simulink library "BLDC_controller_Lib_CounterBased"  (R2025a)
settings: Solver=VariableStepAuto  StartTime=0.0  StopTime=10.0  RelTol=1e-3
undefined symbols (not defined in the file): a_elecAngle, a_elecPeriod, a_phaAdv_M1, b_phaAdvEna, cf_speedCoef, cf_speedFilt, CTRL_COMM, n_commAcvLo, n_commDeacvHi, r_commDCDeacv, r_sin3PhaA_M1, r_sin3PhaB_M1, r_sin3PhaC_M1, r_sinPhaA_M1, r_sinPhaB_M1, r_sinPhaC_M1, r_trapPhaA_M1, r_trapPhaB_M1, r_trapPhaC_M1, vec_hallToPos, z_commutMap_M1, z_ctrlTypSel, z_hallDebSteps, z_maxCntRst, z_nrEdgeSpdAcv
libraries: BLDC_controller_Lib x4, simulink_extras x1, $bdroot x1, simulink x1, BLDC_controller_Lib_new x1
(part 1 of 2)
settings Model: Creator=37ef  LastModifiedBy=ernes
settings SolverCC: AlgebraicLoopSolver=TrustRegion
settings DataIOCC: ReturnWorkspaceOutputs=off
settings DebuggingCC: UnconnectedInputMsg=warning  UnconnectedOutputMsg=warning  UnconnectedLineMsg=warning  ArithmeticOperatorsInVariantConditions=warning
settings ModelReferenceCC: EnableRefExpFcnMdlSchedulingChecks=on
settings SFSimCC: SimUseLocalCustomCode=off  CustomCodeUndefinedFunction=UseInterfaceOnly
settings RTWCC: RTWUseLocalCustomCode=off  GPUComputeCapability=3.5

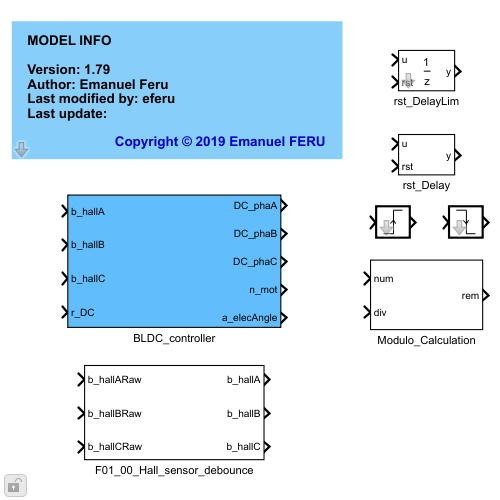
[thumbnail: Simulink's stored preview of the top-level diagram]
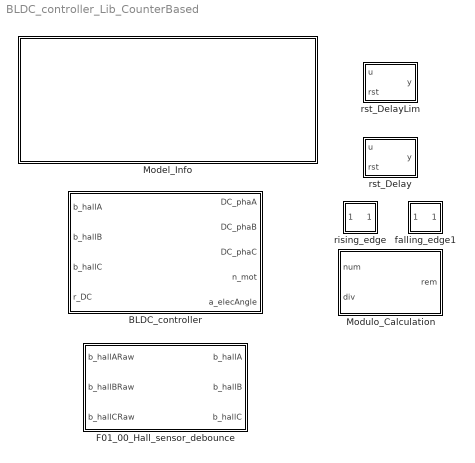
== system BLDC_controller_Lib_CounterBased ==
  BLDC_controller : Subsystem  SystemSampleTime=1e-5
  F01_00_Hall_sensor_debounce : Subsystem
  Model_Info : Subsystem
      mask DialogControl DescGroupVar Prompt: Model info
      mask DialogControl DescTextVar Prompt: This mask gives quick information about the model.
      mask Display:
      | info = Simulink.MDLInfo(bdroot);
      | file = dir([bdroot '.slx']);
      | % image('logo.png', [0.48, 0.55, 0.5, 0.4]);
      | text(0.05, 0.5, [...
      |         'MODEL INFO \n\n' ...
      |         'Version: ' info.ModelVersion '\n' ...
      |         'Author: ' 'Emanuel Feru' '\n' ...
      |         'Last modified by: ' info.LastModifiedBy '\n' ...
      |         'Last update: ' file.date '\n\n'], ...
      |         'horizontalAlignment', 'left', ...
      |         'verticalAlignment', 'middle');
      | 
      | color('blue');
      | text(0.95, 0.08, [...
      |         'Copyright © 2019 Emanuel FERU'], ...
      |         'horizontalAlignment', 'right', ...
      |         'verticalAlignment', 'bottom');
  Modulo_Calculation : Subsystem
  falling_edge1 : Subsystem  StopFcn=%tagged  TreatAsAtomicUnit=on  mask(Falling edge detection){}
      mask help:
      | Falling edge detection for a logic signal.
      | When a falling edge on the input signal is detected, the output switches to 1 during one time step.
      settings: RTWSystemCode=Nonreusable function
      mask Display: plot(0,0,100,100, [20 50 50 80], [90 90 10 10], [40 50 60], [55 45 55] )
  rising_edge : Subsystem  StopFcn=%tagged  TreatAsAtomicUnit=on  mask(Rising edge detection){}
      mask help:
      | Rising edge detection for a logic signal.
      | When a rising edge on the input signal is detected, the output switches to 1 during one time step.
      settings: RTWSystemCode=Nonreusable function
      mask Display: plot(0,0,100,100, [20 50 50 80], [10 10 90 90], [40 50 60], [45 55 45] )
  rst_Delay : Subsystem
  rst_DelayLim : Subsystem  mask{z_cntMaxLim=200}
      mask prompts: z_cntMaxLim "Maximum counter limit"
      mask Display: dpoly(1,[1 0],'z')

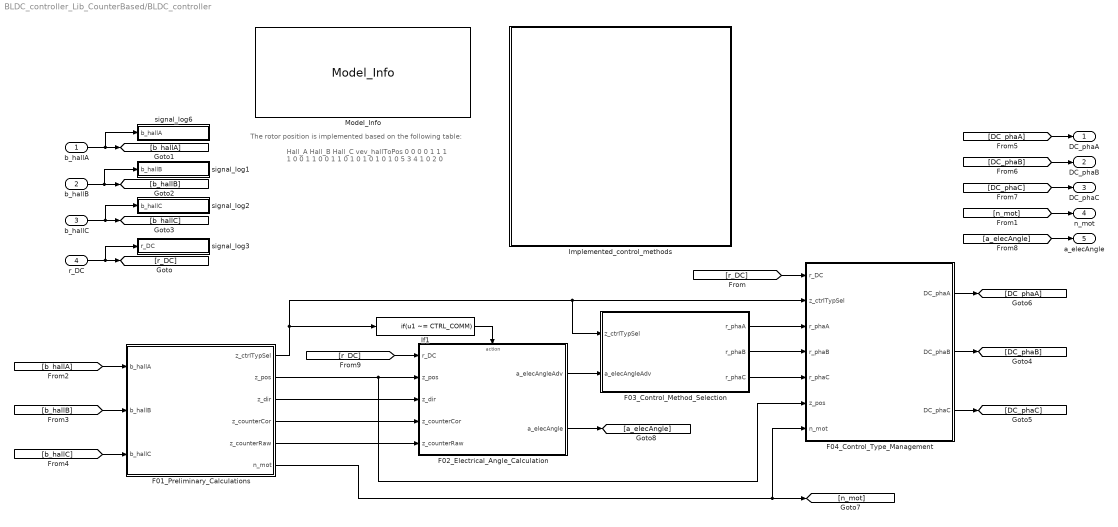
== system BLDC_controller_Lib_CounterBased/BLDC_controller ==
  note: Hall_A
      | Hall_B
      | Hall_C
      | vev_hallToPos
      |
      | 0
      | 0
      | 0
      | 0
      | 1
      | 1
      | 1
      | 1
      | 0
      | 0
      | 1
      | 1
      | 0
      | 0
      | 1
      | 1
      | 0
      | 1
      | 0
      | 1
      | 0
      | 1
      | 0
      | 1
      | 0
      | 5
      | 3
      | 4
      | 1
      | 0
      | 2
      | 0
  note: The rotor position is implemented based on the following table:
  "b_hallA " : Inport
  b_hallB : Inport  Port=2
  b_hallC : Inport  Port=3
  r_DC : Inport  Port=4
  F01_Preliminary_Calculations : Subsystem
  F02_Electrical_Angle_Calculation : Subsystem
  F03_Control_Method_Selection : Subsystem
  F04_Control_Type_Management : Subsystem
  If1 : If  IfExpression=u1 ~= CTRL_COMM  ShowElse=off
  Implemented_control_methods : Subsystem
      mask Display: image('control_methods.png')
  Model_Info : $bdroot/Model_Info
  signal_log1 : Subsystem
  signal_log2 : Subsystem
  signal_log3 : Subsystem
  signal_log6 : Subsystem
  DC_phaA : Outport  VectorParamsAs1DForOutWhenUnconnected=off
  DC_phaB : Outport  Port=2  VectorParamsAs1DForOutWhenUnconnected=off
  DC_phaC : Outport  Port=3  VectorParamsAs1DForOutWhenUnconnected=off
  n_mot : Outport  Port=4  VectorParamsAs1DForOutWhenUnconnected=off
  a_elecAngle : Outport  Port=5  VectorParamsAs1DForOutWhenUnconnected=off
  wires:
  [r_DC] -> F02_Electrical_Angle_Calculation/1(r_DC)
  F02_Electrical_Angle_Calculation/2(a_elecAngle) -> [a_elecAngle]
  [a_elecAngle] -> a_elecAngle/1
  r_DC/1 -> [r_DC], signal_log3/1(r_DC)
  [DC_phaC] -> DC_phaC/1
  [DC_phaB] -> DC_phaB/1
  F04_Control_Type_Management/3("DC_phaC ") -> [DC_phaC]
  F04_Control_Type_Management/2(DC_phaB) -> [DC_phaB]
  F04_Control_Type_Management/1(DC_phaA) -> [DC_phaA]
  [r_DC] -> F04_Control_Type_Management/1(r_DC)
  F03_Control_Method_Selection/3("r_phaC ") -> F04_Control_Type_Management/5(r_phaC)
  F03_Control_Method_Selection/2(r_phaB) -> F04_Control_Type_Management/4(r_phaB)
  F03_Control_Method_Selection/1(r_phaA) -> F04_Control_Type_Management/3(r_phaA)
  F02_Electrical_Angle_Calculation/1(a_elecAngleAdv) -> F03_Control_Method_Selection/2(a_elecAngleAdv)
  If1/1 -> F02_Electrical_Angle_Calculation/Action
  F01_Preliminary_Calculations/1(z_ctrlTypSel) -> If1/1, F03_Control_Method_Selection/1(z_ctrlTypSel), F04_Control_Type_Management/2(z_ctrlTypSel)
  F01_Preliminary_Calculations/5(z_counterRaw) -> F02_Electrical_Angle_Calculation/5(z_counterRaw)
  F01_Preliminary_Calculations/4(z_counterCor) -> F02_Electrical_Angle_Calculation/4(z_counterCor)
  F01_Preliminary_Calculations/6("n_mot ") -> [n_mot], F04_Control_Type_Management/7(n_mot)
  F01_Preliminary_Calculations/3(z_dir) -> F02_Electrical_Angle_Calculation/3(z_dir)
  F01_Preliminary_Calculations/2(z_pos) -> F02_Electrical_Angle_Calculation/2(z_pos), F04_Control_Type_Management/6(z_pos)
  [b_hallB] -> F01_Preliminary_Calculations/2(b_hallB)
  [b_hallC] -> F01_Preliminary_Calculations/3(b_hallC)
  [b_hallA] -> F01_Preliminary_Calculations/1(b_hallA)
  [DC_phaA] -> DC_phaA/1
  [n_mot] -> n_mot/1
  b_hallC/1 -> [b_hallC], signal_log2/1(b_hallC)
  b_hallB/1 -> [b_hallB], signal_log1/1(b_hallB)
  "b_hallA "/1 -> [b_hallA], signal_log6/1(b_hallA)

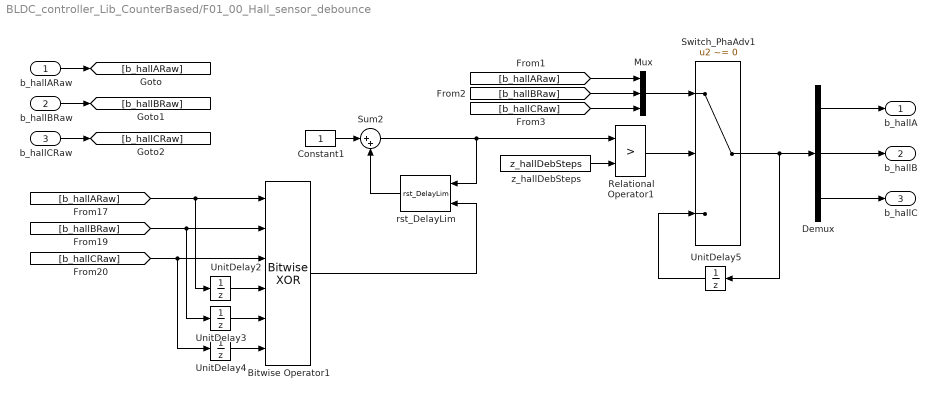
== system BLDC_controller_Lib_CounterBased/F01_00_Hall_sensor_debounce ==
  b_hallARaw : Inport
  b_hallBRaw : Inport  Port=2
  b_hallCRaw : Inport  Port=3
  Bitwise Operator1 : simulink/Logic and Bit Operations/Bitwise Operator  logicop=XOR  UseBitMask=off  NumInputPorts=6  BitMask=bin2dec('11011001')  BitMaskRealWorld=Stored Integer
  Constant1 : Constant  OutDataTypeStr=uint8
  Demux : Demux  Outputs=3
  Mux : Mux  Inputs=3
  Relational Operator1 : RelationalOperator  Operator=>  OutDataTypeStr=boolean  RndMeth=Simplest  InputSameDT=off
  Sum2 : Sum  Inputs=|++  InputSameDT=on  RndMeth=Simplest  OutDataTypeStr=Inherit: Same as first input
  Switch_PhaAdv1 : Switch  Criteria=u2 ~= 0  OutDataTypeStr=Inherit: Inherit via back propagation  RndMeth=Zero  SaturateOnIntegerOverflow=off  InputSameDT=off
  UnitDelay{2..5} (4 alike) : UnitDelay  SampleTime=-1  HasFrameUpgradeWarning=on
  rst_DelayLim : BLDC_controller_Lib_new/rst_DelayLim  z_cntMaxLim=200
  z_hallDebSteps : Constant  Value=z_hallDebSteps  OutDataTypeStr=Inherit: Inherit via back propagation
  b_hallA : Outport  OutputWhenDisabled=reset  InitialOutput=0  VectorParamsAs1DForOutWhenUnconnected=off
  b_hallB : Outport  Port=2  OutputWhenDisabled=reset  InitialOutput=0  VectorParamsAs1DForOutWhenUnconnected=off
  b_hallC : Outport  Port=3  OutputWhenDisabled=reset  InitialOutput=0  VectorParamsAs1DForOutWhenUnconnected=off
  wires:
  [b_hallCRaw] -> Mux/3
  [b_hallBRaw] -> Mux/2
  [b_hallARaw] -> Mux/1
  b_hallCRaw/1 -> [b_hallCRaw]
  b_hallBRaw/1 -> [b_hallBRaw]
  b_hallARaw/1 -> [b_hallARaw]
  [b_hallBRaw] -> UnitDelay3/1, Bitwise Operator1/2
  Demux/2 -> b_hallB/1
  Demux/1 -> b_hallA/1
  Mux/1 -> Switch_PhaAdv1/1
  Demux/3 -> b_hallC/1
  Relational Operator1/1 -> Switch_PhaAdv1/2
  [b_hallARaw] -> UnitDelay2/1, Bitwise Operator1/1
  UnitDelay5/1 -> Switch_PhaAdv1/3
  Switch_PhaAdv1/1 -> Demux/1, UnitDelay5/1
  [b_hallCRaw] -> UnitDelay4/1, Bitwise Operator1/3
  UnitDelay2/1 -> Bitwise Operator1/4
  UnitDelay4/1 -> Bitwise Operator1/6
  UnitDelay3/1 -> Bitwise Operator1/5
  Constant1/1 -> Sum2/1
  rst_DelayLim/1 -> Sum2/2
  z_hallDebSteps/1 -> Relational Operator1/2
  Bitwise Operator1/1 -> rst_DelayLim/2
  Sum2/1 -> rst_DelayLim/1, Relational Operator1/1

== system BLDC_controller_Lib_CounterBased/Model_Info ==

== system BLDC_controller_Lib_CounterBased/Modulo_Calculation ==
  note: Modulo implementation: rem = num - div*(num/div)
      | Note : Division and multiplier has the setting 'Floor'
  num : Inport
  div : Inport  Port=2
  Divide2 : Product  Inputs=*/  OutDataTypeStr=Inherit: Same as first input
  Divide3 : Product  Inputs=**  OutDataTypeStr=Inherit: Same as first input
  Sum3 : Sum  Inputs=|+-  RndMeth=Simplest  OutDataTypeStr=Inherit: Same as first input
  rem : Outport  VectorParamsAs1DForOutWhenUnconnected=off
  wires:
  num/1 -> Sum3/1, Divide2/1
  Sum3/1 -> rem/1
  Divide3/1 -> Sum3/2
  div/1 -> Divide3/2, Divide2/2
  Divide2/1 -> Divide3/1

== system BLDC_controller_Lib_CounterBased/falling_edge1 ==
  Signal : Inport
  Logical Operator : Logic  Tag=struct('inputs','2','comment',struct('text','','placement',1),'logdata',struct('maxnumvals',inf,'plotchannels',[],'loggingmode',3,'channels',1),'operator','AND','output',struct('variable','','description','','name','$S_$B','address','','class','default','type','Bool','unit',''),'scalingvalid',0,'date',733067.68453166669)  OutDataTypeStr=boolean
  Logical Operator1 : Logic  Tag=struct('inputs','1','comment',struct('text','','placement',1),'logdata',struct('maxnumvals',inf,'plotchannels',[],'loggingmode',3,'channels',1),'operator','NOT','output',struct('variable','','description','','name','$S_$B','address','','class','default','type','Bool','unit',''),'scalingvalid',0,'date',733067.68453201384)  Operator=NOT  Inputs=1  OutDataTypeStr=boolean
  UnitDelay : UnitDelay  SampleTime=-1  HasFrameUpgradeWarning=on
      settings: AttributesFormatString=Te = %<SampleTime>\nIni=%<X0>
  Out : Outport  VectorParamsAs1DForOutWhenUnconnected=off
  wires:
  UnitDelay/1 -> Logical Operator/2
  Logical Operator1/1 -> Logical Operator/1
  Signal/1 -> UnitDelay/1, Logical Operator1/1
  Logical Operator/1 -> Out/1

== system BLDC_controller_Lib_CounterBased/rising_edge ==
  Signal : Inport
  Logical Operator : Logic  Tag=struct('inputs','2','comment',struct('text','','placement',1),'logdata',struct('maxnumvals',inf,'plotchannels',[],'loggingmode',3,'channels',1),'operator','AND','output',struct('variable','','description','','name','$S_$B','address','','class','default','type','Bool','unit',''),'scalingvalid',0,'date',733067.68458487268)  OutDataTypeStr=boolean
  Logical Operator1 : Logic  Tag=struct('inputs','1','comment',struct('text','','placement',1),'logdata',struct('maxnumvals',inf,'plotchannels',[],'loggingmode',3,'channels',1),'operator','NOT','output',struct('variable','','description','','name','$S_$B','address','','class','default','type','Bool','unit',''),'scalingvalid',0,'date',733067.68458533566)  Operator=NOT  Inputs=1  OutDataTypeStr=boolean
  UnitDelay : UnitDelay  SampleTime=-1  HasFrameUpgradeWarning=on
      settings: AttributesFormatString=Te = %<SampleTime>\nIni=%<X0>
  Out : Outport  VectorParamsAs1DForOutWhenUnconnected=off
  wires:
  UnitDelay/1 -> Logical Operator1/1
  Logical Operator1/1 -> Logical Operator/2
  Signal/1 -> Logical Operator/1, UnitDelay/1
  Logical Operator/1 -> Out/1

== system BLDC_controller_Lib_CounterBased/rst_Delay ==
  u : Inport
  rst : Inport  Port=2
  Constant23 : Constant  Value=0  OutDataTypeStr=Inherit: Inherit via back propagation
  Switch1 : Switch  Criteria=u2 ~= 0  OutDataTypeStr=Inherit: Inherit via back propagation  RndMeth=Simplest  SaturateOnIntegerOverflow=off  InputSameDT=off
  UnitDelay1 : UnitDelay  SampleTime=-1  HasFrameUpgradeWarning=on
  y : Outport  VectorParamsAs1DForOutWhenUnconnected=off
  wires:
  Switch1/1 -> y/1
  u/1 -> UnitDelay1/1
  UnitDelay1/1 -> Switch1/3
  rst/1 -> Switch1/2
  Constant23/1 -> Switch1/1

== system BLDC_controller_Lib_CounterBased/rst_DelayLim ==
  u : Inport
  rst : Inport  Port=2
  Constant1 : Constant  Value=z_cntMaxLim  OutDataTypeStr=Inherit: Inherit via back propagation
  Constant23 : Constant  Value=0  OutDataTypeStr=Inherit: Inherit via back propagation
  Relational Operator1 : RelationalOperator  Operator=<  OutDataTypeStr=boolean  RndMeth=Simplest  InputSameDT=off
  Switch1 : Switch  Criteria=u2 ~= 0  OutDataTypeStr=Inherit: Inherit via back propagation  RndMeth=Simplest  SaturateOnIntegerOverflow=off  InputSameDT=off
  Switch2 : Switch  Criteria=u2 ~= 0  OutDataTypeStr=Inherit: Inherit via back propagation  RndMeth=Simplest  SaturateOnIntegerOverflow=off  InputSameDT=off
  UnitDelay1 : UnitDelay  InitialCondition=z_cntMaxLim  SampleTime=-1  HasFrameUpgradeWarning=on
  y : Outport  VectorParamsAs1DForOutWhenUnconnected=off
  wires:
  Switch1/1 -> y/1
  u/1 -> UnitDelay1/1
  rst/1 -> Switch1/2
  Constant23/1 -> Switch1/1
  UnitDelay1/1 -> Switch2/1, Relational Operator1/1
  Constant1/1 -> Switch2/3, Relational Operator1/2
  Relational Operator1/1 -> Switch2/2
  Switch2/1 -> Switch1/3

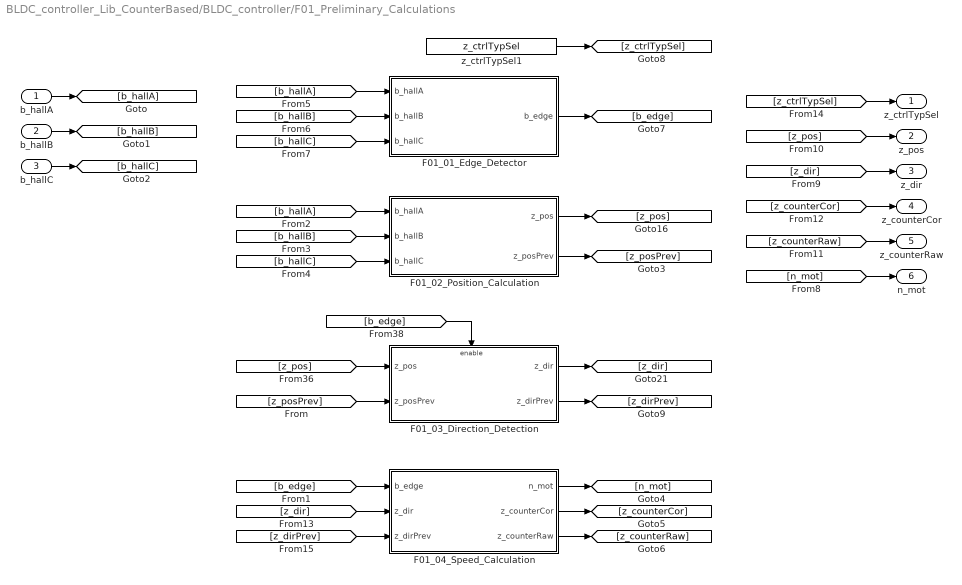
== system BLDC_controller_Lib_CounterBased/BLDC_controller/F01_Preliminary_Calculations ==
  b_hallA : Inport
  b_hallB : Inport  Port=2
  b_hallC : Inport  Port=3
  F01_01_Edge_Detector : Subsystem
  F01_02_Position_Calculation : Subsystem
  F01_03_Direction_Detection : Subsystem
  F01_04_Speed_Calculation : Subsystem
  z_ctrlTypSel1 : Constant  Value=z_ctrlTypSel  OutDataTypeStr=uint8
  z_ctrlTypSel : Outport  OutputWhenDisabled=reset  InitialOutput=0  VectorParamsAs1DForOutWhenUnconnected=off
  z_pos : Outport  Port=2  OutputWhenDisabled=reset  InitialOutput=0  VectorParamsAs1DForOutWhenUnconnected=off
  z_dir : Outport  Port=3  OutputWhenDisabled=reset  InitialOutput=0  VectorParamsAs1DForOutWhenUnconnected=off
  z_counterCor : Outport  Port=4  OutputWhenDisabled=reset  InitialOutput=0  VectorParamsAs1DForOutWhenUnconnected=off
  z_counterRaw : Outport  Port=5  OutputWhenDisabled=reset  InitialOutput=0  VectorParamsAs1DForOutWhenUnconnected=off
  "n_mot " : Outport  Port=6  OutputWhenDisabled=reset  InitialOutput=0  VectorParamsAs1DForOutWhenUnconnected=off
  wires:
  [z_dirPrev] -> F01_04_Speed_Calculation/3(z_dirPrev)
  F01_03_Direction_Detection/2(z_dirPrev) -> [z_dirPrev]
  z_ctrlTypSel1/1 -> [z_ctrlTypSel]
  [z_ctrlTypSel] -> z_ctrlTypSel/1
  [z_dir] -> F01_04_Speed_Calculation/2(z_dir)
  [z_counterRaw] -> z_counterRaw/1
  [z_counterCor] -> z_counterCor/1
  F01_04_Speed_Calculation/3(z_counterRaw) -> [z_counterRaw]
  F01_04_Speed_Calculation/2(z_counterCor) -> [z_counterCor]
  [z_pos] -> z_pos/1
  [z_dir] -> z_dir/1
  [n_mot] -> "n_mot "/1
  F01_04_Speed_Calculation/1(n_mot) -> [n_mot]
  [b_edge] -> F01_04_Speed_Calculation/1(b_edge)
  F01_02_Position_Calculation/2(z_posPrev) -> [z_posPrev]
  F01_02_Position_Calculation/1("z_pos ") -> [z_pos]
  [b_hallA] -> F01_02_Position_Calculation/1(b_hallA)
  [b_hallB] -> F01_02_Position_Calculation/2(b_hallB)
  [b_hallC] -> F01_02_Position_Calculation/3(b_hallC)
  b_hallC/1 -> [b_hallC]
  b_hallB/1 -> [b_hallB]
  b_hallA/1 -> [b_hallA]
  [z_posPrev] -> F01_03_Direction_Detection/2(z_posPrev)
  [b_hallC] -> F01_01_Edge_Detector/3(b_hallC)
  [b_hallB] -> F01_01_Edge_Detector/2(b_hallB)
  F01_03_Direction_Detection/1(z_dir) -> [z_dir]
  [b_edge] -> F01_03_Direction_Detection/Enable
  F01_01_Edge_Detector/1("b_edge ") -> [b_edge]
  [b_hallA] -> F01_01_Edge_Detector/1(b_hallA)
  [z_pos] -> F01_03_Direction_Detection/1(z_pos)

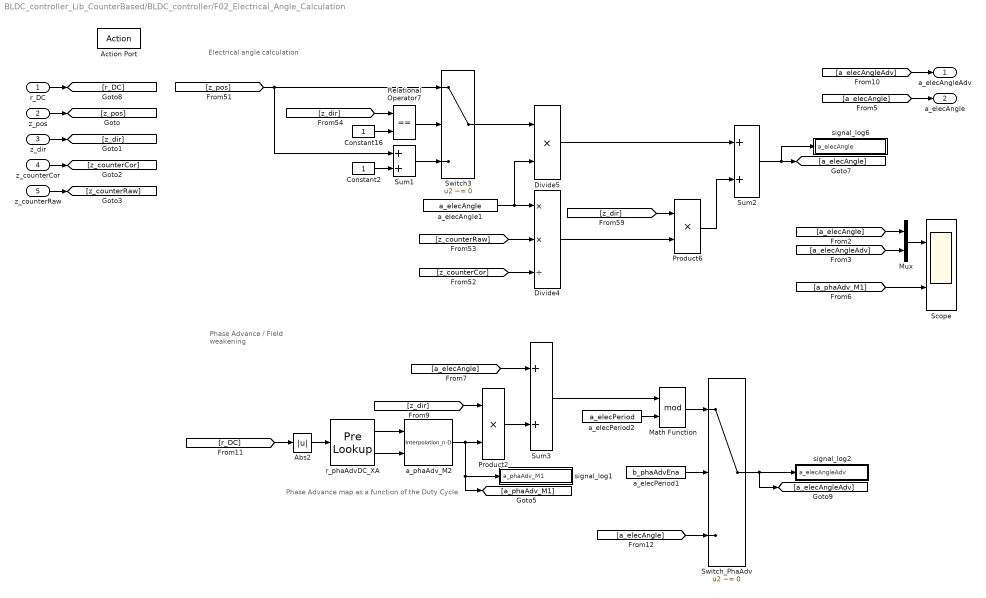
== system BLDC_controller_Lib_CounterBased/BLDC_controller/F02_Electrical_Angle_Calculation ==
  note: Phase Advance map as a function of the Duty Cycle.
  note: Phase Advance / Field weakening
  note: Electrical angle calculation
  r_DC : Inport
  z_pos : Inport  Port=2
  z_dir : Inport  Port=3
  z_counterCor : Inport  Port=4
  z_counterRaw : Inport  Port=5
  Action Port : ActionPort
  Abs2 : Abs  ZeroCross=off  OutDataTypeStr=Inherit: Inherit via back propagation  RndMeth=Simplest  SaturateOnIntegerOverflow=off
  Constant16 : Constant  OutDataTypeStr=Inherit: Inherit via back propagation
  Constant2 : Constant  OutDataTypeStr=Inherit: Inherit via back propagation
  Divide4 : Product  Inputs=**/  OutDataTypeStr=int32  RndMeth=Simplest
  Divide5 : Product  Inputs=**  OutDataTypeStr=int32  RndMeth=Simplest
  Math Function : Math  Operator=mod  SignedPower=on
  Mux : Mux  Inputs=2
  Product2 : Product  RndMeth=Simplest
  Product6 : Product  OutDataTypeStr=Inherit: Inherit via back propagation  RndMeth=Simplest
  Relational Operator7 : RelationalOperator  Operator===  OutDataTypeStr=boolean  RndMeth=Simplest  InputSameDT=off
  Scope : Scope  NumInputPorts=2
      settings: ActiveDisplayYMinimum=-50.125  ActiveDisplayYMaximum=411.125
  Sum1 : Sum  RndMeth=Simplest  OutDataTypeStr=Inherit: Same as first input
  Sum2 : Sum  RndMeth=Simplest  OutDataTypeStr=Inherit: Same as first input
  Sum3 : Sum  RndMeth=Simplest  OutDataTypeStr=Inherit: Same as first input
  Switch3 : Switch  Criteria=u2 ~= 0  OutDataTypeStr=Inherit: Inherit via back propagation  RndMeth=Zero  SaturateOnIntegerOverflow=off  InputSameDT=off
  Switch_PhaAdv : Switch  Criteria=u2 ~= 0  OutDataTypeStr=Inherit: Inherit via back propagation  RndMeth=Zero  SaturateOnIntegerOverflow=off  InputSameDT=off
  a_elecAngle1 : Constant  Value=a_elecAngle  OutDataTypeStr=int32
  a_elecPeriod1 : Constant  Value=b_phaAdvEna  OutDataTypeStr=boolean
  a_elecPeriod2 : Constant  Value=a_elecPeriod  OutDataTypeStr=Inherit: Inherit via back propagation
  a_phaAdv_M2 : Interpolation_n-D  NumberOfTableDimensions=1  Table=a_phaAdv_M1  ExtrapMethod=Clip  OutDataTypeStr=int16  InternalRulePriority=Speed  RndMeth=Simplest
      settings: InputPortMap=u0,u1
  r_phaAdvDC_XA : PreLookup  BreakpointsData=r_phaAdvDC_XA  IndexSearchMethod=Evenly spaced points  IndexDataTypeStr=uint8  RndMeth=Simplest
  signal_log1 : Subsystem
  signal_log2 : Subsystem
  signal_log6 : Subsystem
  a_elecAngleAdv : Outport  OutputWhenDisabled=reset  InitialOutput=0  VectorParamsAs1DForOutWhenUnconnected=off
  a_elecAngle : Outport  Port=2  OutputWhenDisabled=reset  InitialOutput=0  VectorParamsAs1DForOutWhenUnconnected=off
  wires:
  Sum3/1 -> Math Function/1
  Math Function/1 -> Switch_PhaAdv/1
  a_elecPeriod2/1 -> Math Function/2
  Abs2/1 -> r_phaAdvDC_XA/1
  [r_DC] -> Abs2/1
  a_phaAdv_M2/1 -> Product2/2, [a_phaAdv_M1], signal_log1/1(a_phaAdv_M1)
  [a_elecAngle] -> Sum3/1
  Product2/1 -> Sum3/2
  [z_dir] -> Product2/1
  Switch_PhaAdv/1 -> signal_log2/1(a_elecAngleAdv), [a_elecAngleAdv]
  r_DC/1 -> [r_DC]
  [a_elecAngle] -> Switch_PhaAdv/3
  r_phaAdvDC_XA/1 -> a_phaAdv_M2/1
  r_phaAdvDC_XA/2 -> a_phaAdv_M2/2
  a_elecPeriod1/1 -> Switch_PhaAdv/2
  [a_phaAdv_M1] -> Scope/2
  [a_elecAngleAdv] -> a_elecAngleAdv/1
  [a_elecAngle] -> a_elecAngle/1
  Divide4/1 -> Product6/2
  [z_dir] -> Product6/1
  Sum1/1 -> Switch3/3
  [a_elecAngleAdv] -> Mux/2
  [a_elecAngle] -> Mux/1
  Mux/1 -> Scope/1
  Sum2/1 -> [a_elecAngle], signal_log6/1(a_elecAngle)
  Constant2/1 -> Sum1/2
  z_counterRaw/1 -> [z_counterRaw]
  a_elecAngle1/1 -> Divide5/2, Divide4/1
  [z_counterRaw] -> Divide4/2
  Constant16/1 -> Relational Operator7/2
  Divide5/1 -> Sum2/1
  [z_dir] -> Relational Operator7/1
  Product6/1 -> Sum2/2
  Relational Operator7/1 -> Switch3/2
  [z_pos] -> Switch3/1, Sum1/1
  [z_counterCor] -> Divide4/3
  Switch3/1 -> Divide5/1
  z_counterCor/1 -> [z_counterCor]
  z_dir/1 -> [z_dir]
  z_pos/1 -> [z_pos]

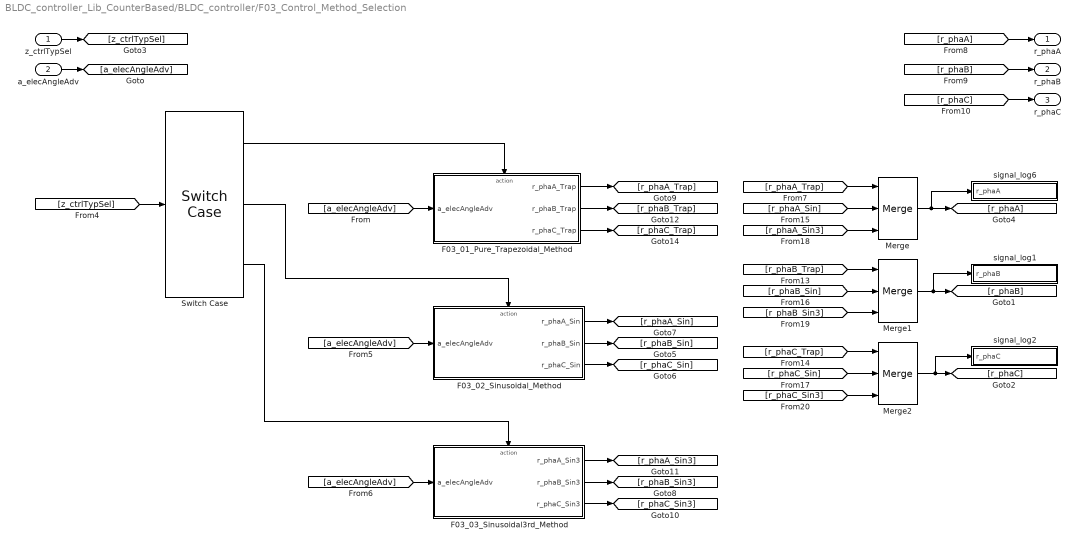
== system BLDC_controller_Lib_CounterBased/BLDC_controller/F03_Control_Method_Selection ==
  z_ctrlTypSel : Inport
  a_elecAngleAdv : Inport  Port=2
  F03_01_Pure_Trapezoidal_Method : Subsystem
  F03_02_Sinusoidal_Method : Subsystem
  F03_03_Sinusoidal3rd_Method : Subsystem
  Merge : Merge  Inputs=3
  Merge1 : Merge  Inputs=3
  Merge2 : Merge  Inputs=3
  Switch Case : SwitchCase  CaseConditions={CTRL_TRAP, CTRL_SIN, CTRL_SIN3}  ShowDefaultCase=off
  signal_log1 : Subsystem
  signal_log2 : Subsystem
  signal_log6 : Subsystem
  r_phaA : Outport  OutputWhenDisabled=reset  InitialOutput=0  VectorParamsAs1DForOutWhenUnconnected=off
  r_phaB : Outport  Port=2  OutputWhenDisabled=reset  InitialOutput=0  VectorParamsAs1DForOutWhenUnconnected=off
  "r_phaC " : Outport  Port=3  OutputWhenDisabled=reset  InitialOutput=0  VectorParamsAs1DForOutWhenUnconnected=off
  wires:
  [r_phaC_Sin3] -> Merge2/3
  [r_phaC_Sin] -> Merge2/2
  [r_phaB_Sin3] -> Merge1/3
  [r_phaC_Trap] -> Merge2/1
  [r_phaB_Sin] -> Merge1/2
  [r_phaB_Trap] -> Merge1/1
  [r_phaA_Sin3] -> Merge/3
  [r_phaA_Sin] -> Merge/2
  z_ctrlTypSel/1 -> [z_ctrlTypSel]
  [r_phaA_Trap] -> Merge/1
  Merge2/1 -> [r_phaC], signal_log2/1(r_phaC)
  Merge1/1 -> [r_phaB], signal_log1/1(r_phaB)
  Merge/1 -> [r_phaA], signal_log6/1(r_phaA)
  F03_03_Sinusoidal3rd_Method/1(r_phaA_Sin3) -> [r_phaA_Sin3]
  F03_03_Sinusoidal3rd_Method/2(r_phaB_Sin3) -> [r_phaB_Sin3]
  F03_03_Sinusoidal3rd_Method/3(r_phaC_Sin3) -> [r_phaC_Sin3]
  F03_02_Sinusoidal_Method/1(r_phaA_Sin) -> [r_phaA_Sin]
  F03_02_Sinusoidal_Method/2(r_phaB_Sin) -> [r_phaB_Sin]
  F03_02_Sinusoidal_Method/3(r_phaC_Sin) -> [r_phaC_Sin]
  F03_01_Pure_Trapezoidal_Method/3(r_phaC_Trap) -> [r_phaC_Trap]
  F03_01_Pure_Trapezoidal_Method/2(r_phaB_Trap) -> [r_phaB_Trap]
  Switch Case/3 -> F03_03_Sinusoidal3rd_Method/Action
  Switch Case/2 -> F03_02_Sinusoidal_Method/Action
  [a_elecAngleAdv] -> F03_03_Sinusoidal3rd_Method/1(a_elecAngleAdv)
  [a_elecAngleAdv] -> F03_02_Sinusoidal_Method/1(a_elecAngleAdv)
  Switch Case/1 -> F03_01_Pure_Trapezoidal_Method/Action
  [a_elecAngleAdv] -> F03_01_Pure_Trapezoidal_Method/1(a_elecAngleAdv)
  [z_ctrlTypSel] -> Switch Case/1
  F03_01_Pure_Trapezoidal_Method/1(r_phaA_Trap) -> [r_phaA_Trap]
  a_elecAngleAdv/1 -> [a_elecAngleAdv]
  [r_phaC] -> "r_phaC "/1
  [r_phaB] -> r_phaB/1
  [r_phaA] -> r_phaA/1

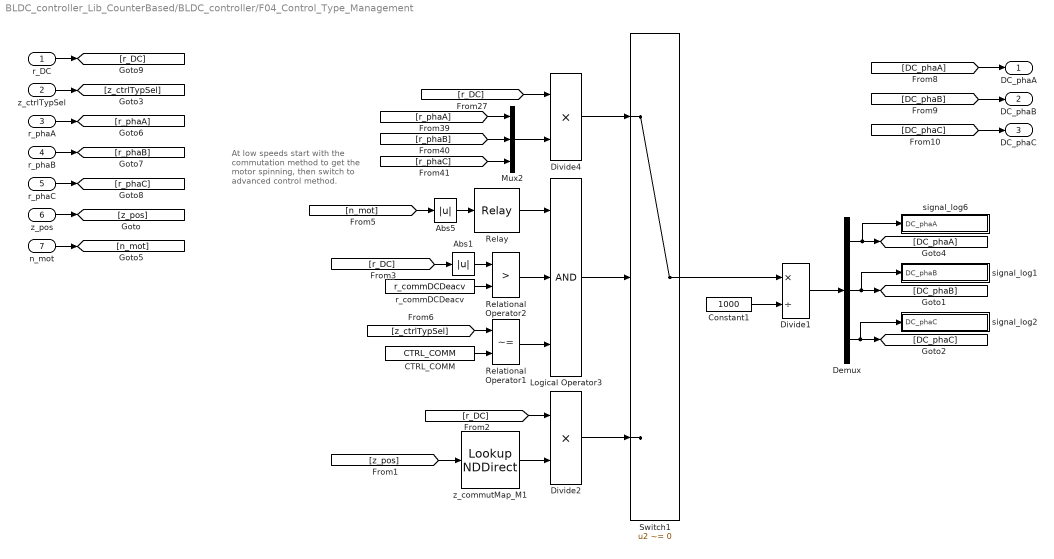
== system BLDC_controller_Lib_CounterBased/BLDC_controller/F04_Control_Type_Management ==
  note: At low speeds start with the commutation method to get the motor spinning, then switch to advanced control method.
  r_DC : Inport
  z_ctrlTypSel : Inport  Port=2
  r_phaA : Inport  Port=3
  r_phaB : Inport  Port=4
  r_phaC : Inport  Port=5
  z_pos : Inport  Port=6
  n_mot : Inport  Port=7
  Abs1 : Abs  OutDataTypeStr=Inherit: Inherit via back propagation  RndMeth=Zero  SaturateOnIntegerOverflow=off
  Abs5 : Abs  OutDataTypeStr=Inherit: Inherit via back propagation  RndMeth=Zero  SaturateOnIntegerOverflow=off
  CTRL_COMM : Constant  Value=CTRL_COMM  OutDataTypeStr=Inherit: Inherit via back propagation
  Constant1 : Constant  Value=1000  OutDataTypeStr=Inherit: Inherit via back propagation
  Demux : Demux  Outputs=3
  Divide1 : Product  Inputs=*/  RndMeth=Simplest  OutDataTypeStr=Inherit: Same as first input
  Divide2 : Product  Inputs=**  RndMeth=Simplest  OutDataTypeStr=Inherit: Same as first input
  Divide4 : Product  Inputs=**  RndMeth=Simplest  OutDataTypeStr=Inherit: Same as first input
  Logical Operator3 : Logic  Inputs=3  AllPortsSameDT=off  OutDataTypeStr=boolean
  Mux2 : Mux  Inputs=3
  Relational Operator1 : RelationalOperator  Operator=~=  OutDataTypeStr=boolean  RndMeth=Simplest  InputSameDT=off
  Relational Operator2 : RelationalOperator  Operator=>  OutDataTypeStr=boolean  RndMeth=Simplest  InputSameDT=off
  Relay : Relay  OnSwitchValue=n_commDeacvHi  OffSwitchValue=n_commAcvLo  OutDataTypeStr=boolean
  Switch1 : Switch  Criteria=u2 ~= 0  OutDataTypeStr=Inherit: Inherit via back propagation  RndMeth=Zero  SaturateOnIntegerOverflow=off  InputSameDT=off
  r_commDCDeacv : Constant  Value=r_commDCDeacv  OutDataTypeStr=Inherit: Inherit via back propagation
  signal_log1 : Subsystem
  signal_log2 : Subsystem
  signal_log6 : Subsystem
  z_commutMap_M1 : LookupNDDirect  InputsSelectThisObjectFromTable=Vector  Table=z_commutMap_M1  DiagnosticForOutOfRangeInput=None  TableDataTypeStr=int16
  DC_phaA : Outport  OutputWhenDisabled=reset  InitialOutput=0  VectorParamsAs1DForOutWhenUnconnected=off
  DC_phaB : Outport  Port=2  OutputWhenDisabled=reset  InitialOutput=0  VectorParamsAs1DForOutWhenUnconnected=off
  "DC_phaC " : Outport  Port=3  OutputWhenDisabled=reset  InitialOutput=0  VectorParamsAs1DForOutWhenUnconnected=off
  wires:
  Abs1/1 -> Relational Operator2/1
  Relational Operator2/1 -> Logical Operator3/2
  Relational Operator1/1 -> Logical Operator3/3
  r_commDCDeacv/1 -> Relational Operator2/2
  [r_DC] -> Abs1/1
  [r_DC] -> Divide4/1
  Logical Operator3/1 -> Switch1/2
  [n_mot] -> Abs5/1
  Divide2/1 -> Switch1/3
  z_commutMap_M1/1 -> Divide2/2
  [r_DC] -> Divide2/1
  Constant1/1 -> Divide1/2
  Divide4/1 -> Switch1/1
  Mux2/1 -> Divide4/2
  [r_phaC] -> Mux2/3
  [r_phaB] -> Mux2/2
  [r_phaA] -> Mux2/1
  r_DC/1 -> [r_DC]
  r_phaC/1 -> [r_phaC]
  r_phaB/1 -> [r_phaB]
  r_phaA/1 -> [r_phaA]
  n_mot/1 -> [n_mot]
  Divide1/1 -> Demux/1
  [z_pos] -> z_commutMap_M1/1
  Abs5/1 -> Relay/1
  CTRL_COMM/1 -> Relational Operator1/2
  [z_ctrlTypSel] -> Relational Operator1/1
  Relay/1 -> Logical Operator3/1
  Switch1/1 -> Divide1/1
  [DC_phaA] -> DC_phaA/1
  [DC_phaB] -> DC_phaB/1
  [DC_phaC] -> "DC_phaC "/1
  z_pos/1 -> [z_pos]
  Demux/1 -> [DC_phaA], signal_log6/1(DC_phaA)
  Demux/2 -> signal_log1/1(DC_phaB), [DC_phaB]
  Demux/3 -> signal_log2/1(DC_phaC), [DC_phaC]
  z_ctrlTypSel/1 -> [z_ctrlTypSel]

== system BLDC_controller_Lib_CounterBased/BLDC_controller/Implemented_control_methods ==

== system BLDC_controller_Lib_CounterBased/BLDC_controller/signal_log1 ==
  b_hallB : Inport
  Terminator_1 : Terminator
  wires:
  b_hallB/1 -> Terminator_1/1  "b_hallB"

== system BLDC_controller_Lib_CounterBased/BLDC_controller/signal_log2 ==
  b_hallC : Inport
  Terminator_1 : Terminator
  wires:
  b_hallC/1 -> Terminator_1/1  "b_hallC"

== system BLDC_controller_Lib_CounterBased/BLDC_controller/signal_log3 ==
  r_DC : Inport
  Terminator_1 : Terminator
  wires:
  r_DC/1 -> Terminator_1/1  "r_DC"

== system BLDC_controller_Lib_CounterBased/BLDC_controller/signal_log6 ==
  b_hallA : Inport
  Terminator_1 : Terminator
  wires:
  b_hallA/1 -> Terminator_1/1  "b_hallA"

== system BLDC_controller_Lib_CounterBased/BLDC_controller/F01_Preliminary_Calculations/F01_01_Edge_Detector ==
  b_hallA : Inport
  b_hallB : Inport  Port=2
  b_hallC : Inport  Port=3
  Logical Operator : Logic  Operator=XOR  Inputs=6  AllPortsSameDT=off  OutDataTypeStr=boolean
  UnitDelay : UnitDelay  SampleTime=-1  HasFrameUpgradeWarning=on
  UnitDelay1 : UnitDelay  SampleTime=-1  HasFrameUpgradeWarning=on
  UnitDelay2 : UnitDelay  SampleTime=-1  HasFrameUpgradeWarning=on
  signal_log6 : Subsystem
  "b_edge " : Outport  OutputWhenDisabled=reset  InitialOutput=0  VectorParamsAs1DForOutWhenUnconnected=off
  wires:
  UnitDelay/1 -> Logical Operator/4
  UnitDelay2/1 -> Logical Operator/6
  UnitDelay1/1 -> Logical Operator/5
  Logical Operator/1 -> signal_log6/1(b_edge), "b_edge "/1
  b_hallB/1 -> Logical Operator/2, UnitDelay1/1
  b_hallC/1 -> Logical Operator/3, UnitDelay2/1
  b_hallA/1 -> Logical Operator/1, UnitDelay/1

== system BLDC_controller_Lib_CounterBased/BLDC_controller/F01_Preliminary_Calculations/F01_02_Position_Calculation ==
  note: This calculates the low resolution position based on Hall sensors.
  b_hallA : Inport
  b_hallB : Inport  Port=2
  b_hallC : Inport  Port=3
  Selector : Selector  IndexMode=Zero-based  InputPortWidth=length(vec_hallToPos)  IndexOptions=Index vector (port)  Indices=[1 3]  OutputSizes=1
  Sum : Sum  Inputs=+++  RndMeth=Simplest  OutDataTypeStr=Inherit: Same as first input
  UnitDelay1 : UnitDelay  SampleTime=-1  HasFrameUpgradeWarning=on
  g_Ha : Gain  Gain=4  OutDataTypeStr=Inherit: Inherit via back propagation  RndMeth=Zero  ParamDataTypeStr=Inherit: Same as input
  g_Hb : Gain  Gain=2  OutDataTypeStr=Inherit: Inherit via back propagation  RndMeth=Simplest  ParamDataTypeStr=Inherit: Same as input
  signal_log6 : Subsystem
  vec_hallToPos : Constant  Value=vec_hallToPos  OutDataTypeStr=uint8
  "z_pos " : Outport  OutputWhenDisabled=reset  InitialOutput=0  VectorParamsAs1DForOutWhenUnconnected=off
  z_posPrev : Outport  Port=2  OutputWhenDisabled=reset  InitialOutput=0  VectorParamsAs1DForOutWhenUnconnected=off
  wires:
  Selector/1 -> signal_log6/1(z_pos), UnitDelay1/1, "z_pos "/1
  UnitDelay1/1 -> z_posPrev/1
  vec_hallToPos/1 -> Selector/1
  b_hallB/1 -> g_Hb/1
  b_hallA/1 -> g_Ha/1
  Sum/1 -> Selector/2
  g_Hb/1 -> Sum/2
  g_Ha/1 -> Sum/1
  b_hallC/1 -> Sum/3

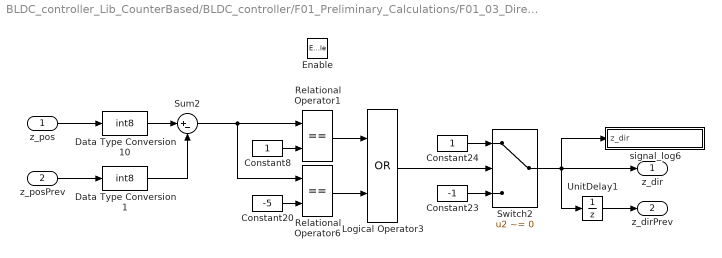
== system BLDC_controller_Lib_CounterBased/BLDC_controller/F01_Preliminary_Calculations/F01_03_Direction_Detection ==
  z_pos : Inport
  z_posPrev : Inport  Port=2
  Enable : EnablePort  ZeroCross=off
  Constant20 : Constant  Value=-5  OutDataTypeStr=Inherit: Inherit via back propagation
  Constant23 : Constant  Value=-1  OutDataTypeStr=int8
  Constant24 : Constant  OutDataTypeStr=int8
  Constant8 : Constant  OutDataTypeStr=Inherit: Inherit via back propagation
  Data Type Conversion1 : DataTypeConversion  OutDataTypeStr=int8  SaturateOnIntegerOverflow=off  RndMeth=Floor
  Data Type Conversion10 : DataTypeConversion  OutDataTypeStr=int8  SaturateOnIntegerOverflow=off  RndMeth=Floor
  Logical Operator3 : Logic  Operator=OR  AllPortsSameDT=off  OutDataTypeStr=boolean
  Relational Operator1 : RelationalOperator  Operator===  OutDataTypeStr=boolean  RndMeth=Simplest  InputSameDT=off
  Relational Operator6 : RelationalOperator  Operator===  OutDataTypeStr=boolean  RndMeth=Simplest  InputSameDT=off
  Sum2 : Sum  Inputs=|+-  InputSameDT=on  RndMeth=Zero  OutDataTypeStr=Inherit: Same as first input
  Switch2 : Switch  Criteria=u2 ~= 0  OutDataTypeStr=Inherit: Inherit via back propagation  RndMeth=Simplest  SaturateOnIntegerOverflow=off  InputSameDT=off
  UnitDelay1 : UnitDelay  SampleTime=-1  HasFrameUpgradeWarning=on
  signal_log6 : Subsystem
  z_dir : Outport  VectorParamsAs1DForOutWhenUnconnected=off
  z_dirPrev : Outport  Port=2  VectorParamsAs1DForOutWhenUnconnected=off
  wires:
  UnitDelay1/1 -> z_dirPrev/1
  Data Type Conversion1/1 -> Sum2/2
  Data Type Conversion10/1 -> Sum2/1
  Switch2/1 -> UnitDelay1/1, signal_log6/1(z_dir), z_dir/1
  Logical Operator3/1 -> Switch2/2
  Constant23/1 -> Switch2/3
  Constant24/1 -> Switch2/1
  Constant20/1 -> Relational Operator6/2
  Relational Operator6/1 -> Logical Operator3/2
  Sum2/1 -> Relational Operator1/1, Relational Operator6/1
  Constant8/1 -> Relational Operator1/2
  Relational Operator1/1 -> Logical Operator3/1
  z_posPrev/1 -> Data Type Conversion1/1
  z_pos/1 -> Data Type Conversion10/1

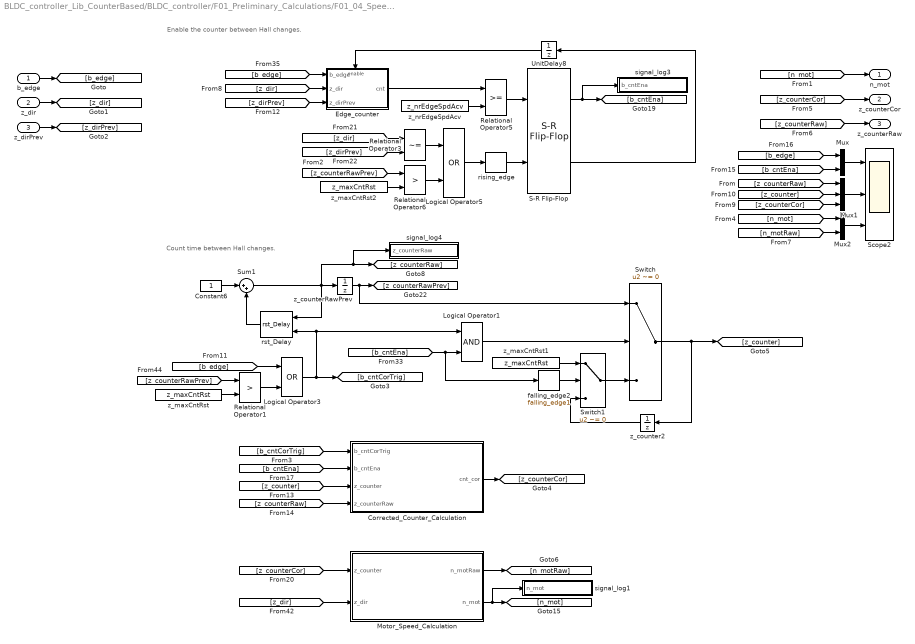
== system BLDC_controller_Lib_CounterBased/BLDC_controller/F01_Preliminary_Calculations/F01_04_Speed_Calculation ==
  note: Enable the counter between Hall changes.
  note: Count time between Hall changes.
  b_edge : Inport
  z_dir : Inport  Port=2
  z_dirPrev : Inport  Port=3
  Constant6 : Constant  OutDataTypeStr=Inherit: Inherit via back propagation
  Corrected_Counter_Calculation : Subsystem
  Edge_counter : Subsystem
  Logical Operator1 : Logic  AllPortsSameDT=off  OutDataTypeStr=boolean
  Logical Operator3 : Logic  Operator=OR  AllPortsSameDT=off  OutDataTypeStr=boolean
  Logical Operator5 : Logic  Operator=OR  AllPortsSameDT=off  OutDataTypeStr=boolean
  Motor_Speed_Calculation : Subsystem
  Mux : Mux  Inputs=2
  Mux1 : Mux  Inputs=3
  Mux2 : Mux  Inputs=2
  Relational Operator1 : RelationalOperator  Operator=>  OutDataTypeStr=boolean  RndMeth=Simplest  InputSameDT=off
  Relational Operator3 : RelationalOperator  Operator=~=  OutDataTypeStr=boolean  RndMeth=Simplest  InputSameDT=off
  Relational Operator5 : RelationalOperator  OutDataTypeStr=boolean  RndMeth=Simplest  InputSameDT=off
  Relational Operator6 : RelationalOperator  Operator=>  OutDataTypeStr=boolean  RndMeth=Simplest  InputSameDT=off
  S-R Flip-Flop : simulink_extras/Flip Flops/S-R Flip-Flop  initial_condition=0
  Scope2 : Scope  NumInputPorts=3
      settings: ActiveDisplayYMinimum=-0.125  ActiveDisplayYMaximum=1.125
  Sum1 : Sum  Inputs=|++  InputSameDT=on  RndMeth=Simplest  OutDataTypeStr=Inherit: Same as first input
  Switch : Switch  Criteria=u2 ~= 0  OutDataTypeStr=Inherit: Inherit via back propagation  RndMeth=Simplest  SaturateOnIntegerOverflow=off  InputSameDT=off
  Switch1 : Switch  Criteria=u2 ~= 0  OutDataTypeStr=Inherit: Inherit via back propagation  RndMeth=Simplest  SaturateOnIntegerOverflow=off  InputSameDT=off
  UnitDelay8 : UnitDelay  SampleTime=-1  HasFrameUpgradeWarning=on
  falling_edge2 : BLDC_controller_Lib/falling_edge1
  rising_edge : BLDC_controller_Lib/rising_edge  mask(Rising edge detection){}
  rst_Delay : BLDC_controller_Lib/rst_Delay  initVal=0
  signal_log1 : Subsystem
  signal_log3 : Subsystem
  signal_log4 : Subsystem
  z_counter2 : UnitDelay  InitialCondition=z_maxCntRst  SampleTime=-1  HasFrameUpgradeWarning=on
  z_counterRawPrev : UnitDelay  SampleTime=-1  HasFrameUpgradeWarning=on
  z_maxCntRst : Constant  Value=z_maxCntRst  OutDataTypeStr=int16
  z_maxCntRst1 : Constant  Value=z_maxCntRst  OutDataTypeStr=int16
  z_maxCntRst2 : Constant  Value=z_maxCntRst  OutDataTypeStr=int16
  z_nrEdgeSpdAcv : Constant  Value=z_nrEdgeSpdAcv  OutDataTypeStr=Inherit: Inherit via back propagation
  n_mot : Outport  VectorParamsAs1DForOutWhenUnconnected=off
  z_counterCor : Outport  Port=2  VectorParamsAs1DForOutWhenUnconnected=off
  z_counterRaw : Outport  Port=3  VectorParamsAs1DForOutWhenUnconnected=off
  wires:
  S-R Flip-Flop/2 -> UnitDelay8/1
  [z_dirPrev] -> Edge_counter/3(z_dirPrev)
  [z_dir] -> Edge_counter/2(z_dir)
  Relational Operator3/1 -> Logical Operator5/1
  Switch/1 -> [z_counter], z_counter2/1
  Edge_counter/1(cnt) -> Relational Operator5/1
  [b_edge] -> Edge_counter/1(b_edge)
  rising_edge/1 -> S-R Flip-Flop/2
  UnitDelay8/1 -> Edge_counter/Enable
  S-R Flip-Flop/1 -> signal_log3/1(b_cntEna), [b_cntEna]
  z_nrEdgeSpdAcv/1 -> Relational Operator5/2
  Relational Operator5/1 -> S-R Flip-Flop/1
  rst_Delay/1 -> Sum1/2
  z_dirPrev/1 -> [z_dirPrev]
  z_dir/1 -> [z_dir]
  [z_counterRaw] -> z_counterRaw/1
  [z_counterCor] -> z_counterCor/1
  [n_mot] -> n_mot/1
  b_edge/1 -> [b_edge]
  Sum1/1 -> [z_counterRaw], signal_log4/1(z_counterRaw), z_counterRawPrev/1, rst_Delay/1
  Constant6/1 -> Sum1/1
  z_maxCntRst/1 -> Relational Operator1/2
  [z_counterCor] -> Motor_Speed_Calculation/1(z_counter)
  Logical Operator3/1 -> [b_cntCorTrig], rst_Delay/2, Logical Operator1/1
  [b_cntEna] -> Logical Operator1/2, falling_edge2/1
  [z_dir] -> Motor_Speed_Calculation/2(z_dir)
  z_counterRawPrev/1 -> Switch/1, [z_counterRawPrev]
  z_counter2/1 -> Switch1/3
  [z_counterRawPrev] -> Relational Operator1/1
  Relational Operator1/1 -> Logical Operator3/2
  Mux/1 -> Scope2/1
  [b_edge] -> Mux/1
  [b_cntEna] -> Mux/2
  [z_counter] -> Mux1/2
  [z_counterRaw] -> Mux1/1
  Mux1/1 -> Scope2/2
  falling_edge2/1 -> Switch1/2
  [z_dirPrev] -> Relational Operator3/2
  [z_dir] -> Relational Operator3/1
  z_maxCntRst1/1 -> Switch1/1
  Switch1/1 -> Switch/3
  [b_edge] -> Logical Operator3/1
  [z_counterRawPrev] -> Relational Operator6/1
  z_maxCntRst2/1 -> Relational Operator6/2
  Relational Operator6/1 -> Logical Operator5/2
  Logical Operator5/1 -> rising_edge/1
  Motor_Speed_Calculation/2(n_mot) -> signal_log1/1(n_mot), [n_mot]
  [n_mot] -> Mux2/1
  Mux2/1 -> Scope2/3
  [z_counterCor] -> Mux1/3
  [b_cntCorTrig] -> Corrected_Counter_Calculation/1(b_cntCorTrig)
  [z_counter] -> Corrected_Counter_Calculation/3(z_counter)
  [z_counterRaw] -> Corrected_Counter_Calculation/4(z_counterRaw)
  [b_cntEna] -> Corrected_Counter_Calculation/2(b_cntEna)
  Logical Operator1/1 -> Switch/2
  Motor_Speed_Calculation/1(n_motRaw) -> [n_motRaw]
  Corrected_Counter_Calculation/1(cnt_cor) -> [z_counterCor]
  [n_motRaw] -> Mux2/2

== system BLDC_controller_Lib_CounterBased/BLDC_controller/F02_Electrical_Angle_Calculation/signal_log1 ==
  a_phaAdv_M1 : Inport
  Terminator_1 : Terminator
  wires:
  a_phaAdv_M1/1 -> Terminator_1/1  "a_phaAdv_M1"

== system BLDC_controller_Lib_CounterBased/BLDC_controller/F02_Electrical_Angle_Calculation/signal_log2 ==
  a_elecAngleAdv : Inport
  Terminator_1 : Terminator
  wires:
  a_elecAngleAdv/1 -> Terminator_1/1  "a_elecAngleAdv"

== system BLDC_controller_Lib_CounterBased/BLDC_controller/F02_Electrical_Angle_Calculation/signal_log6 ==
  a_elecAngle : Inport
  Terminator_1 : Terminator
  wires:
  a_elecAngle/1 -> Terminator_1/1  "a_elecAngle"

== system BLDC_controller_Lib_CounterBased/BLDC_controller/F03_Control_Method_Selection/F03_01_Pure_Trapezoidal_Method ==
  a_elecAngleAdv : Inport
  Action Port : ActionPort  InitializeStates=reset
  a_trapElecAngle_XA : PreLookup  BreakpointsData=a_trapElecAngle_XA  IndexSearchMethod=Evenly spaced points  IndexDataTypeStr=uint8  RndMeth=Simplest
  r_trapPhaA_M1 : Interpolation_n-D  NumberOfTableDimensions=1  Table=r_trapPhaA_M1  ExtrapMethod=Clip  RemoveProtectionIndex=on  OutDataTypeStr=int16  InternalRulePriority=Speed  RndMeth=Simplest
      settings: InputPortMap=u0,u1
  r_trapPhaB_M1 : Interpolation_n-D  NumberOfTableDimensions=1  Table=r_trapPhaB_M1  ExtrapMethod=Clip  RemoveProtectionIndex=on  OutDataTypeStr=int16  InternalRulePriority=Speed  RndMeth=Simplest
      settings: InputPortMap=u0,u1
  r_trapPhaC_M1 : Interpolation_n-D  NumberOfTableDimensions=1  Table=r_trapPhaC_M1  ExtrapMethod=Clip  RemoveProtectionIndex=on  OutDataTypeStr=int16  InternalRulePriority=Speed  RndMeth=Simplest
      settings: InputPortMap=u0,u1
  r_phaA_Trap : Outport  VectorParamsAs1DForOutWhenUnconnected=off
  r_phaB_Trap : Outport  Port=2  VectorParamsAs1DForOutWhenUnconnected=off
  r_phaC_Trap : Outport  Port=3  VectorParamsAs1DForOutWhenUnconnected=off
  wires:
  a_elecAngleAdv/1 -> a_trapElecAngle_XA/1
  r_trapPhaC_M1/1 -> r_phaC_Trap/1
  r_trapPhaB_M1/1 -> r_phaB_Trap/1
  r_trapPhaA_M1/1 -> r_phaA_Trap/1
  a_trapElecAngle_XA/2 -> r_trapPhaA_M1/2, r_trapPhaB_M1/2, r_trapPhaC_M1/2
  a_trapElecAngle_XA/1 -> r_trapPhaB_M1/1, r_trapPhaC_M1/1, r_trapPhaA_M1/1

== system BLDC_controller_Lib_CounterBased/BLDC_controller/F03_Control_Method_Selection/F03_02_Sinusoidal_Method ==
  a_elecAngleAdv : Inport
  Action Port : ActionPort  InitializeStates=reset
  a_sinElecAngle_XA : PreLookup  BreakpointsData=a_sinElecAngle_XA  IndexSearchMethod=Evenly spaced points  BeginIndexSearchUsingPreviousIndexResult=on  IndexDataTypeStr=uint8  RndMeth=Simplest
  r_sinPhaA_M1 : Interpolation_n-D  NumberOfTableDimensions=1  Table=r_sinPhaA_M1  ExtrapMethod=Clip  RemoveProtectionIndex=on  OutDataTypeStr=int16  InternalRulePriority=Speed  RndMeth=Simplest
      settings: InputPortMap=u0,u1
  r_sinPhaB_M1 : Interpolation_n-D  NumberOfTableDimensions=1  Table=r_sinPhaB_M1  ExtrapMethod=Clip  RemoveProtectionIndex=on  OutDataTypeStr=int16  InternalRulePriority=Speed  RndMeth=Simplest
      settings: InputPortMap=u0,u1
  r_sinPhaC_M1 : Interpolation_n-D  NumberOfTableDimensions=1  Table=r_sinPhaC_M1  ExtrapMethod=Clip  RemoveProtectionIndex=on  OutDataTypeStr=int16  InternalRulePriority=Speed  RndMeth=Simplest
      settings: InputPortMap=u0,u1
  r_phaA_Sin : Outport  VectorParamsAs1DForOutWhenUnconnected=off
  r_phaB_Sin : Outport  Port=2  VectorParamsAs1DForOutWhenUnconnected=off
  r_phaC_Sin : Outport  Port=3  VectorParamsAs1DForOutWhenUnconnected=off
  wires:
  a_sinElecAngle_XA/1 -> r_sinPhaA_M1/1, r_sinPhaC_M1/1, r_sinPhaB_M1/1
  a_sinElecAngle_XA/2 -> r_sinPhaC_M1/2, r_sinPhaB_M1/2, r_sinPhaA_M1/2
  r_sinPhaA_M1/1 -> r_phaA_Sin/1
  r_sinPhaB_M1/1 -> r_phaB_Sin/1
  r_sinPhaC_M1/1 -> r_phaC_Sin/1
  a_elecAngleAdv/1 -> a_sinElecAngle_XA/1

== system BLDC_controller_Lib_CounterBased/BLDC_controller/F03_Control_Method_Selection/F03_03_Sinusoidal3rd_Method ==
  a_elecAngleAdv : Inport
  Action Port : ActionPort  InitializeStates=reset
  a_sinElecAngle_XA : PreLookup  BreakpointsData=a_sinElecAngle_XA  IndexSearchMethod=Evenly spaced points  BeginIndexSearchUsingPreviousIndexResult=on  IndexDataTypeStr=uint8  RndMeth=Simplest
  r_sin3PhaA_M1 : Interpolation_n-D  NumberOfTableDimensions=1  Table=r_sin3PhaA_M1  ExtrapMethod=Clip  RemoveProtectionIndex=on  OutDataTypeStr=int16  InternalRulePriority=Speed  RndMeth=Simplest
      settings: InputPortMap=u0,u1
  r_sin3PhaB_M1 : Interpolation_n-D  NumberOfTableDimensions=1  Table=r_sin3PhaB_M1  ExtrapMethod=Clip  RemoveProtectionIndex=on  OutDataTypeStr=int16  InternalRulePriority=Speed  RndMeth=Simplest
      settings: InputPortMap=u0,u1
  r_sin3PhaC_M1 : Interpolation_n-D  NumberOfTableDimensions=1  Table=r_sin3PhaC_M1  ExtrapMethod=Clip  RemoveProtectionIndex=on  OutDataTypeStr=int16  InternalRulePriority=Speed  RndMeth=Simplest
      settings: InputPortMap=u0,u1
  r_phaA_Sin3 : Outport  VectorParamsAs1DForOutWhenUnconnected=off
  r_phaB_Sin3 : Outport  Port=2  VectorParamsAs1DForOutWhenUnconnected=off
  r_phaC_Sin3 : Outport  Port=3  VectorParamsAs1DForOutWhenUnconnected=off
  wires:
  a_elecAngleAdv/1 -> a_sinElecAngle_XA/1
  r_sin3PhaC_M1/1 -> r_phaC_Sin3/1
  r_sin3PhaB_M1/1 -> r_phaB_Sin3/1
  r_sin3PhaA_M1/1 -> r_phaA_Sin3/1
  a_sinElecAngle_XA/2 -> r_sin3PhaA_M1/2, r_sin3PhaB_M1/2, r_sin3PhaC_M1/2
  a_sinElecAngle_XA/1 -> r_sin3PhaB_M1/1, r_sin3PhaC_M1/1, r_sin3PhaA_M1/1

== system BLDC_controller_Lib_CounterBased/BLDC_controller/F03_Control_Method_Selection/signal_log1 ==
  r_phaB : Inport
  Terminator_1 : Terminator
  wires:
  r_phaB/1 -> Terminator_1/1  "r_phaB"

== system BLDC_controller_Lib_CounterBased/BLDC_controller/F03_Control_Method_Selection/signal_log2 ==
  r_phaC : Inport
  Terminator_1 : Terminator
  wires:
  r_phaC/1 -> Terminator_1/1  "r_phaC"

== system BLDC_controller_Lib_CounterBased/BLDC_controller/F03_Control_Method_Selection/signal_log6 ==
  r_phaA : Inport
  Terminator_1 : Terminator
  wires:
  r_phaA/1 -> Terminator_1/1  "r_phaA"

== system BLDC_controller_Lib_CounterBased/BLDC_controller/F04_Control_Type_Management/signal_log1 ==
  DC_phaB : Inport
  Terminator_1 : Terminator
  wires:
  DC_phaB/1 -> Terminator_1/1  "DC_phaB"

== system BLDC_controller_Lib_CounterBased/BLDC_controller/F04_Control_Type_Management/signal_log2 ==
  DC_phaC : Inport
  Terminator_1 : Terminator
  wires:
  DC_phaC/1 -> Terminator_1/1  "DC_phaC"

== system BLDC_controller_Lib_CounterBased/BLDC_controller/F04_Control_Type_Management/signal_log6 ==
  DC_phaA : Inport
  Terminator_1 : Terminator
  wires:
  DC_phaA/1 -> Terminator_1/1  "DC_phaA"

== system BLDC_controller_Lib_CounterBased/BLDC_controller/F01_Preliminary_Calculations/F01_01_Edge_Detector/signal_log6 ==
  b_edge : Inport
  Terminator_1 : Terminator
  wires:
  b_edge/1 -> Terminator_1/1  "b_edge"

== system BLDC_controller_Lib_CounterBased/BLDC_controller/F01_Preliminary_Calculations/F01_02_Position_Calculation/signal_log6 ==
  z_pos : Inport
  Terminator_1 : Terminator
  wires:
  z_pos/1 -> Terminator_1/1  "z_pos"

== system BLDC_controller_Lib_CounterBased/BLDC_controller/F01_Preliminary_Calculations/F01_03_Direction_Detection/signal_log6 ==
  z_dir : Inport
  Terminator_1 : Terminator
  wires:
  z_dir/1 -> Terminator_1/1  "z_dir"

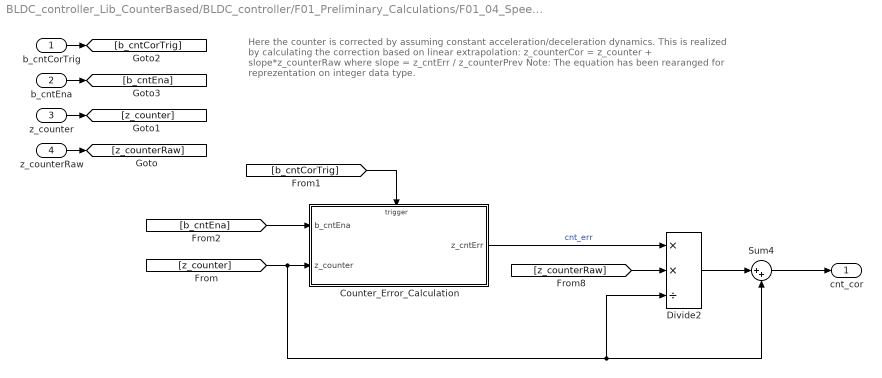
== system BLDC_controller_Lib_CounterBased/BLDC_controller/F01_Preliminary_Calculations/F01_04_Speed_Calculation/Corrected_Counter_Calculation ==
  note: Here the counter is corrected by assuming constant acceleration/deceleration dynamics.
      | This is realized by calculating the correction based on linear extrapolation:
      |
      | z_counterCor = z_counter + slope*z_counterRaw
      | where slope = z_cntErr / z_counterPrev
      |
      | Note: The equation has been rearanged for reprezentation on integer data type.
  b_cntCorTrig : Inport
  b_cntEna : Inport  Port=2
  z_counter : Inport  Port=3
  z_counterRaw : Inport  Port=4
  Counter_Error_Calculation : Subsystem
  Divide2 : Product  Inputs=**/  RndMeth=Simplest  SaturateOnIntegerOverflow=on  OutDataTypeStr=Inherit: Same as first input
  Sum4 : Sum  Inputs=|++  InputSameDT=on  RndMeth=Simplest  OutDataTypeStr=Inherit: Same as first input
  cnt_cor : Outport  VectorParamsAs1DForOutWhenUnconnected=off
  wires:
  [b_cntCorTrig] -> Counter_Error_Calculation/Trigger
  Divide2/1 -> Sum4/1
  [z_counter] -> Divide2/3, Sum4/2, Counter_Error_Calculation/2(z_counter)
  Counter_Error_Calculation/1(z_cntErr) -> Divide2/1  "cnt_err"
  [z_counterRaw] -> Divide2/2
  z_counterRaw/1 -> [z_counterRaw]
  [b_cntEna] -> Counter_Error_Calculation/1(b_cntEna)
  Sum4/1 -> cnt_cor/1
  z_counter/1 -> [z_counter]
  b_cntCorTrig/1 -> [b_cntCorTrig]
  b_cntEna/1 -> [b_cntEna]

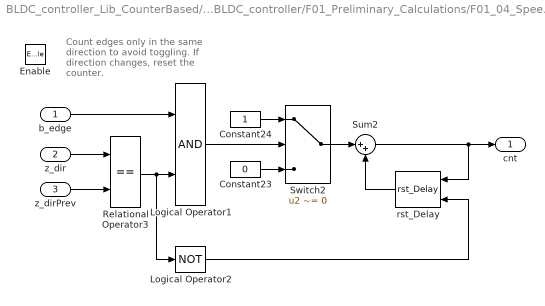
== system BLDC_controller_Lib_CounterBased/BLDC_controller/F01_Preliminary_Calculations/F01_04_Speed_Calculation/Edge_counter ==
  note: Count edges only in the same direction to avoid toggling. If direction changes, reset the counter.
  b_edge : Inport
  z_dir : Inport  Port=2
  z_dirPrev : Inport  Port=3
  Enable : EnablePort  StatesWhenEnabling=reset
  Constant23 : Constant  Value=0  OutDataTypeStr=uint8
  Constant24 : Constant  OutDataTypeStr=uint8
  Logical Operator1 : Logic  AllPortsSameDT=off  OutDataTypeStr=boolean
  Logical Operator2 : Logic  Operator=NOT  AllPortsSameDT=off  OutDataTypeStr=boolean
  Relational Operator3 : RelationalOperator  Operator===  OutDataTypeStr=boolean  RndMeth=Simplest  InputSameDT=off
  Sum2 : Sum  Inputs=|++  InputSameDT=on  OutDataTypeStr=Inherit: Same as first input
  Switch2 : Switch  Criteria=u2 ~= 0  OutDataTypeStr=Inherit: Inherit via back propagation  RndMeth=Simplest  SaturateOnIntegerOverflow=off  InputSameDT=off
  rst_Delay : BLDC_controller_Lib/rst_Delay  initVal=0
  cnt : Outport  OutputWhenDisabled=reset  InitialOutput=0  VectorParamsAs1DForOutWhenUnconnected=off
  wires:
  z_dirPrev/1 -> Relational Operator3/2
  z_dir/1 -> Relational Operator3/1
  Relational Operator3/1 -> Logical Operator1/2, Logical Operator2/1
  Logical Operator2/1 -> rst_Delay/2
  Logical Operator1/1 -> Switch2/2
  b_edge/1 -> Logical Operator1/1
  rst_Delay/1 -> Sum2/2
  Constant24/1 -> Switch2/1
  Constant23/1 -> Switch2/3
  Switch2/1 -> Sum2/1
  Sum2/1 -> cnt/1, rst_Delay/1

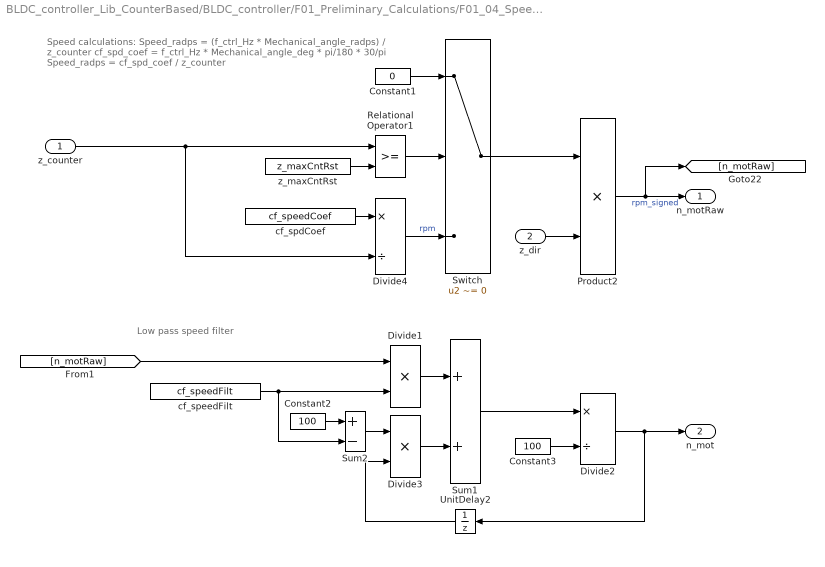
== system BLDC_controller_Lib_CounterBased/BLDC_controller/F01_Preliminary_Calculations/F01_04_Speed_Calculation/Motor_Speed_Calculation ==
  note: Low pass speed filter
  note: Speed calculations:
      | Speed_radps = (f_ctrl_Hz * Mechanical_angle_radps) / z_counter
      | cf_spd_coef = f_ctrl_Hz * Mechanical_angle_deg * pi/180 * 30/pi
      | Speed_radps = cf_spd_coef / z_counter
  z_counter : Inport
  z_dir : Inport  Port=2
  Constant1 : Constant  Value=0  OutDataTypeStr=Inherit: Inherit via back propagation
  Constant2 : Constant  Value=100  OutDataTypeStr=Inherit: Inherit via back propagation
  Constant3 : Constant  Value=100  OutDataTypeStr=Inherit: Inherit via back propagation
  Divide1 : Product  Inputs=**  RndMeth=Simplest  OutDataTypeStr=Inherit: Same as first input
  Divide2 : Product  Inputs=*/  RndMeth=Simplest  OutDataTypeStr=Inherit: Same as first input
  Divide3 : Product  Inputs=**  RndMeth=Simplest  OutDataTypeStr=Inherit: Same as first input
  Divide4 : Product  Inputs=*/  RndMeth=Simplest  OutDataTypeStr=Inherit: Same as first input
  Product2 : Product  RndMeth=Simplest  OutDataTypeStr=Inherit: Same as first input
  Relational Operator1 : RelationalOperator  OutDataTypeStr=boolean  RndMeth=Simplest  InputSameDT=off
  Sum1 : Sum  InputSameDT=on  RndMeth=Simplest  OutDataTypeStr=Inherit: Same as first input
  Sum2 : Sum  Inputs=+-  InputSameDT=on  RndMeth=Simplest  OutDataTypeStr=Inherit: Same as first input
  Switch : Switch  Criteria=u2 ~= 0  OutDataTypeStr=Inherit: Inherit via back propagation  RndMeth=Simplest  SaturateOnIntegerOverflow=off  InputSameDT=off
  UnitDelay2 : UnitDelay  SampleTime=-1  HasFrameUpgradeWarning=on
  cf_spdCoef : Constant  Value=cf_speedCoef  OutDataTypeStr=int32
  cf_speedFilt : Constant  Value=cf_speedFilt  OutDataTypeStr=int32
  z_maxCntRst : Constant  Value=z_maxCntRst  OutDataTypeStr=Inherit: Inherit via back propagation
  n_motRaw : Outport  VectorParamsAs1DForOutWhenUnconnected=off
  n_mot : Outport  Port=2  VectorParamsAs1DForOutWhenUnconnected=off
  wires:
  [n_motRaw] -> Divide1/1
  cf_speedFilt/1 -> Divide1/2, Sum2/2
  Sum2/1 -> Divide3/1
  Constant2/1 -> Sum2/1
  Divide3/1 -> Sum1/2
  z_maxCntRst/1 -> Relational Operator1/2
  Product2/1 -> n_motRaw/1, [n_motRaw]  "rpm_signed"
  z_dir/1 -> Product2/2
  Constant1/1 -> Switch/1
  cf_spdCoef/1 -> Divide4/1
  Relational Operator1/1 -> Switch/2
  Switch/1 -> Product2/1
  Divide4/1 -> Switch/3  "rpm"
  z_counter/1 -> Relational Operator1/1, Divide4/2
  UnitDelay2/1 -> Divide3/2
  Divide1/1 -> Sum1/1
  Divide2/1 -> n_mot/1, UnitDelay2/1
  Sum1/1 -> Divide2/1
  Constant3/1 -> Divide2/2

== system BLDC_controller_Lib_CounterBased/BLDC_controller/F01_Preliminary_Calculations/F01_04_Speed_Calculation/signal_log1 ==
  n_mot : Inport
  Terminator_1 : Terminator
  wires:
  n_mot/1 -> Terminator_1/1  "n_mot"

== system BLDC_controller_Lib_CounterBased/BLDC_controller/F01_Preliminary_Calculations/F01_04_Speed_Calculation/signal_log3 ==
  b_cntEna : Inport
  Terminator_1 : Terminator
  wires:
  b_cntEna/1 -> Terminator_1/1  "b_cntEna"

== system BLDC_controller_Lib_CounterBased/BLDC_controller/F01_Preliminary_Calculations/F01_04_Speed_Calculation/signal_log4 ==
  z_counterRaw : Inport
  Terminator_1 : Terminator
  wires:
  z_counterRaw/1 -> Terminator_1/1  "z_counterRaw"
